simulink model "Model_14Bus_Microgrid_paper_Latam"  (R2022b)
settings: Solver=VariableStepAuto  StartTime=0.0  StopTime=0.5  MaxStep=1e-2  RelTol=1e-3
InitFcn:
  | Set_parameters_R2018
StopFcn:
  | %Save_Data;
  | %Graphics_mod;
values from neighbouring files (symbols this model uses):
  Clink = Ceq*2    (= 0.217013888889)    [Set_parameters.m]
  dis1 = 0.15    [Set_parameters.m]
  dis10 = 6    [Set_parameters.m]
  dis11 = 3    [Set_parameters.m]
  dis12 = 6    [Set_parameters.m]
  dis13 = 3    [Set_parameters.m]
  dis14 = 2    [Set_parameters.m]
  dis2 = 0.2    [Set_parameters.m]
  dis3 = 0.15    [Set_parameters.m]
  dis4 = 0.4    [Set_parameters.m]
  dis5 = 0.4    [Set_parameters.m]
  dis6 = 0.4    [Set_parameters.m]
  dis7 = 0.1    [Set_parameters.m]
  dis8 = 2    [Set_parameters.m]
  dis9 = 6    [Set_parameters.m]
  Fc = 33 * Fnom    (= 1980)    [Set_parameters.m]
  Fnom = 60    [Set_parameters.m]
  Increment_MPPT = 0.01    [Set_parameters.m]
  Ki_Ireg = 20    [Set_parameters.m]
  Ki_VDCreg = 400    [Set_parameters.m]
  Kp_Ireg = 0.3    [Set_parameters.m]
  Kp_VDCreg = 2    [Set_parameters.m]
  LimitL_Ireg = -1.5    [Set_parameters.m]
  LimitL_VDCreg = -1.5    [Set_parameters.m]
  Limits_MPPT = [ 583 357 ]    [Set_parameters.m]
  LimitU_Ireg = 1.5    [Set_parameters.m]
  LimitU_VDCreg = 1.5    [Set_parameters.m]
  P_Load_2 = S_Load_2* PF_Load_2    (= 36000)    [Set_parameters.m]
  P_Load_3 = S_Load_3* PF_Load_3    (= 25500)    [Set_parameters.m]
  Pnom = 1e6    (= 1000000)    [Set_parameters.m]
  Pnom_T1 = 1.5e6    (= 1500000)    [Set_parameters.m]
  Pnom_T2 = 1.5e6    (= 1500000)    [Set_parameters.m]
  Pnom_T3 = 4e6    (= 4000000)    [Set_parameters.m]
  Pnom_xfo = Pnom    (= 1000000)    [Set_parameters.m]
  Ql_Load_2 = S_Load_2 * sin(acos(PF_Load_2))    [Set_parameters.m]
  Ql_Load_3 = S_Load_3 * sin(acos(PF_Load_3))    [Set_parameters.m]
  R_Load_9 = (Vnom_prim * 1.35)^2 / P_Load_9    (= 1084.6153125)    [Set_parameters.m]
  R_Load_DC = Vnom_DC^2/ P_Load_DC    (= 45)    [Set_parameters.m]
  Rl = 0.394    [Set_parameters.m]
  Rls = 0.198    [Set_parameters.m]
  Ts = Ts_Power    (= 5.05050505051e-06)    [Set_parameters.m]
  Ts_Control = 10*Ts_Power    (= 5.05050505051e-05)    [Set_parameters.m]
  Ts_Power = 1/(33*Fnom)/100    (= 5.05050505051e-06)    [Set_parameters.m]
  V1_LL_T3 = 69e3    (= 69000)    [Set_parameters.m]
  Vf = 0    [Set_parameters.m]
  Vfd = 0    [Set_parameters.m]
  Vnom_dc = 480    [Set_parameters.m]
  Vnom_Diesel = 2.4e3    (= 2400)    [Set_parameters.m]
  Vnom_prim = 13.8e3    (= 13800)    [Set_parameters.m]
  Vnom_sec = 220    [Set_parameters.m]
  Vnom_ter_AC_DC = 150    [Set_parameters.m]
  Xl = 0.1168    [Set_parameters.m]
  Xls = 0.1089    [Set_parameters.m]
undefined symbols (not defined in the file or in its folder): D1, Delta, DiscIntNeverNeededParam, Hydride, Ion, level, Lithium, max_min, Metal, Nickel, RL, RLff, sigbuilder_block
libraries: spsRMSLib x73, powerlib_extras x53, spsCurrentMeasurementLib x47, spsTHDLib x26, spsThreePhaseVIMeasurementLib x25, spsVoltageMeasurementLib x23, spsSeriesRLCBranchLib x21, spsThreePhaseSeriesRLCBranchLib x21, spsIGBTDiodeLib x15, spsThreePhaseBreakerLib x14, spsPowerLib x14, spsThreePhaseTransformerTwoWindingsLib x12
(part 8 of 10)

== system Model_14Bus_Microgrid_paper_Latam/Bus_9/PLL/Pll3 ==
  note: error
  note: d'
  note: Fundamental
  note: fase
      | total
  note: fase de la señal
  note: adelanta 90
  note: Este PLL calcula la fase respecto a una onda coseno
  señal : Inport
  w : Inport  Port=2
  Gain : Gain  Gain=-1  SaturateOnIntegerOverflow=on  OutDataTypeStr=Inherit: Same as input  ParamDataTypeStr=Inherit: Same as input
  Integrator : Integrator  InitialCondition=2*pi*60
  Integrator1 : Integrator  InitialCondition=2*pi*60
  Integrator2 : Integrator
  K : Gain  Gain=100  SaturateOnIntegerOverflow=on  OutDataTypeStr=Inherit: Same as input  ParamDataTypeStr=Inherit: Same as input
  Kp : Gain  Gain=10  SaturateOnIntegerOverflow=on  OutDataTypeStr=Inherit: Same as input  ParamDataTypeStr=Inherit: Same as input
  Kp1 : Gain  Gain=10  SaturateOnIntegerOverflow=on  OutDataTypeStr=Inherit: Same as input  ParamDataTypeStr=Inherit: Same as input
  Poduct : Product  SaturateOnIntegerOverflow=on  OutDataTypeStr=Inherit: Same as first input
  Poduct1 : Product  SaturateOnIntegerOverflow=on  OutDataTypeStr=Inherit: Same as first input
  Poduct2 : Product  SaturateOnIntegerOverflow=on  OutDataTypeStr=Inherit: Same as first input
  Sum : Sum  Inputs=|+-  SaturateOnIntegerOverflow=on
  Sum1 : Sum  SaturateOnIntegerOverflow=on
  Sum2 : Sum  Inputs=|-+  SaturateOnIntegerOverflow=on
  Trigonometric Function : Trigonometry
  Trigonometric Function1 : Trigonometry  Operator=cos
  f cos (rad) : Outport  VectorParamsAs1DForOutWhenUnconnected=off
  wires:
  Sum/1 -> Poduct/1, Poduct1/1
  Poduct/1 -> Kp/1
  Kp/1 -> Kp1/1
  Poduct2/1 -> Sum/2
  Trigonometric Function1/1 -> Poduct1/2, Poduct2/1
  Poduct1/1 -> K/1
  K/1 -> Integrator2/1
  Integrator2/1 -> Poduct2/2
  Integrator/1 -> Trigonometric Function/1, Sum2/2, Trigonometric Function1/1
  Integrator1/1 -> Sum2/1
  Sum2/1 -> f cos (rad)/1
  w/1 -> Sum1/1, Integrator1/1
  Kp1/1 -> Sum1/2
  Sum1/1 -> Integrator/1
  Trigonometric Function/1 -> Gain/1
  Gain/1 -> Poduct/2
  señal/1 -> Sum/1

== system Model_14Bus_Microgrid_paper_Latam/Bus_slack /PLL/Pll1 ==
  note: error
  note: d'
  note: Fundamental
  note: fase
      | total
  note: fase de la señal
  note: adelanta 90
  note: Este PLL calcula la fase respecto a una onda coseno
  señal : Inport
  w : Inport  Port=2
  Gain : Gain  Gain=-1  SaturateOnIntegerOverflow=on  OutDataTypeStr=Inherit: Same as input  ParamDataTypeStr=Inherit: Same as input
  Integrator : Integrator  InitialCondition=2*pi*60
  Integrator1 : Integrator  InitialCondition=2*pi*60
  Integrator2 : Integrator
  K : Gain  Gain=100  SaturateOnIntegerOverflow=on  OutDataTypeStr=Inherit: Same as input  ParamDataTypeStr=Inherit: Same as input
  Kp : Gain  Gain=10  SaturateOnIntegerOverflow=on  OutDataTypeStr=Inherit: Same as input  ParamDataTypeStr=Inherit: Same as input
  Kp1 : Gain  Gain=10  SaturateOnIntegerOverflow=on  OutDataTypeStr=Inherit: Same as input  ParamDataTypeStr=Inherit: Same as input
  Poduct : Product  SaturateOnIntegerOverflow=on  OutDataTypeStr=Inherit: Same as first input
  Poduct1 : Product  SaturateOnIntegerOverflow=on  OutDataTypeStr=Inherit: Same as first input
  Poduct2 : Product  SaturateOnIntegerOverflow=on  OutDataTypeStr=Inherit: Same as first input
  Sum : Sum  Inputs=|+-  SaturateOnIntegerOverflow=on
  Sum1 : Sum  SaturateOnIntegerOverflow=on
  Sum2 : Sum  Inputs=|-+  SaturateOnIntegerOverflow=on
  Trigonometric Function : Trigonometry
  Trigonometric Function1 : Trigonometry  Operator=cos
  f cos (rad) : Outport  VectorParamsAs1DForOutWhenUnconnected=off
  wires:
  Sum/1 -> Poduct/1, Poduct1/1
  Poduct/1 -> Kp/1
  Kp/1 -> Kp1/1
  Poduct2/1 -> Sum/2
  Trigonometric Function1/1 -> Poduct1/2, Poduct2/1
  Poduct1/1 -> K/1
  K/1 -> Integrator2/1
  Integrator2/1 -> Poduct2/2
  Integrator/1 -> Trigonometric Function/1, Sum2/2, Trigonometric Function1/1
  Integrator1/1 -> Sum2/1
  Sum2/1 -> f cos (rad)/1
  w/1 -> Sum1/1, Integrator1/1
  Kp1/1 -> Sum1/2
  Sum1/1 -> Integrator/1
  Trigonometric Function/1 -> Gain/1
  Gain/1 -> Poduct/2
  señal/1 -> Sum/1

== system Model_14Bus_Microgrid_paper_Latam/Bus_slack /PLL/Pll2 ==
  note: error
  note: d'
  note: Fundamental
  note: fase
      | total
  note: fase de la señal
  note: adelanta 90
  note: Este PLL calcula la fase respecto a una onda coseno
  señal : Inport
  w : Inport  Port=2
  Gain : Gain  Gain=-1  SaturateOnIntegerOverflow=on  OutDataTypeStr=Inherit: Same as input  ParamDataTypeStr=Inherit: Same as input
  Integrator : Integrator  InitialCondition=2*pi*60
  Integrator1 : Integrator  InitialCondition=2*pi*60
  Integrator2 : Integrator
  K : Gain  Gain=100  SaturateOnIntegerOverflow=on  OutDataTypeStr=Inherit: Same as input  ParamDataTypeStr=Inherit: Same as input
  Kp : Gain  Gain=10  SaturateOnIntegerOverflow=on  OutDataTypeStr=Inherit: Same as input  ParamDataTypeStr=Inherit: Same as input
  Kp1 : Gain  Gain=10  SaturateOnIntegerOverflow=on  OutDataTypeStr=Inherit: Same as input  ParamDataTypeStr=Inherit: Same as input
  Poduct : Product  SaturateOnIntegerOverflow=on  OutDataTypeStr=Inherit: Same as first input
  Poduct1 : Product  SaturateOnIntegerOverflow=on  OutDataTypeStr=Inherit: Same as first input
  Poduct2 : Product  SaturateOnIntegerOverflow=on  OutDataTypeStr=Inherit: Same as first input
  Sum : Sum  Inputs=|+-  SaturateOnIntegerOverflow=on
  Sum1 : Sum  SaturateOnIntegerOverflow=on
  Sum2 : Sum  Inputs=|-+  SaturateOnIntegerOverflow=on
  Trigonometric Function : Trigonometry
  Trigonometric Function1 : Trigonometry  Operator=cos
  f cos (rad) : Outport  VectorParamsAs1DForOutWhenUnconnected=off
  wires:
  Sum/1 -> Poduct/1, Poduct1/1
  Poduct/1 -> Kp/1
  Kp/1 -> Kp1/1
  Poduct2/1 -> Sum/2
  Trigonometric Function1/1 -> Poduct1/2, Poduct2/1
  Poduct1/1 -> K/1
  K/1 -> Integrator2/1
  Integrator2/1 -> Poduct2/2
  Integrator/1 -> Trigonometric Function/1, Sum2/2, Trigonometric Function1/1
  Integrator1/1 -> Sum2/1
  Sum2/1 -> f cos (rad)/1
  w/1 -> Sum1/1, Integrator1/1
  Kp1/1 -> Sum1/2
  Sum1/1 -> Integrator/1
  Trigonometric Function/1 -> Gain/1
  Gain/1 -> Poduct/2
  señal/1 -> Sum/1

== system Model_14Bus_Microgrid_paper_Latam/Bus_slack /PLL/Pll3 ==
  note: error
  note: d'
  note: Fundamental
  note: fase
      | total
  note: fase de la señal
  note: adelanta 90
  note: Este PLL calcula la fase respecto a una onda coseno
  señal : Inport
  w : Inport  Port=2
  Gain : Gain  Gain=-1  SaturateOnIntegerOverflow=on  OutDataTypeStr=Inherit: Same as input  ParamDataTypeStr=Inherit: Same as input
  Integrator : Integrator  InitialCondition=2*pi*60
  Integrator1 : Integrator  InitialCondition=2*pi*60
  Integrator2 : Integrator
  K : Gain  Gain=100  SaturateOnIntegerOverflow=on  OutDataTypeStr=Inherit: Same as input  ParamDataTypeStr=Inherit: Same as input
  Kp : Gain  Gain=10  SaturateOnIntegerOverflow=on  OutDataTypeStr=Inherit: Same as input  ParamDataTypeStr=Inherit: Same as input
  Kp1 : Gain  Gain=10  SaturateOnIntegerOverflow=on  OutDataTypeStr=Inherit: Same as input  ParamDataTypeStr=Inherit: Same as input
  Poduct : Product  SaturateOnIntegerOverflow=on  OutDataTypeStr=Inherit: Same as first input
  Poduct1 : Product  SaturateOnIntegerOverflow=on  OutDataTypeStr=Inherit: Same as first input
  Poduct2 : Product  SaturateOnIntegerOverflow=on  OutDataTypeStr=Inherit: Same as first input
  Sum : Sum  Inputs=|+-  SaturateOnIntegerOverflow=on
  Sum1 : Sum  SaturateOnIntegerOverflow=on
  Sum2 : Sum  Inputs=|-+  SaturateOnIntegerOverflow=on
  Trigonometric Function : Trigonometry
  Trigonometric Function1 : Trigonometry  Operator=cos
  f cos (rad) : Outport  VectorParamsAs1DForOutWhenUnconnected=off
  wires:
  Sum/1 -> Poduct/1, Poduct1/1
  Poduct/1 -> Kp/1
  Kp/1 -> Kp1/1
  Poduct2/1 -> Sum/2
  Trigonometric Function1/1 -> Poduct1/2, Poduct2/1
  Poduct1/1 -> K/1
  K/1 -> Integrator2/1
  Integrator2/1 -> Poduct2/2
  Integrator/1 -> Trigonometric Function/1, Sum2/2, Trigonometric Function1/1
  Integrator1/1 -> Sum2/1
  Sum2/1 -> f cos (rad)/1
  w/1 -> Sum1/1, Integrator1/1
  Kp1/1 -> Sum1/2
  Sum1/1 -> Integrator/1
  Trigonometric Function/1 -> Gain/1
  Gain/1 -> Poduct/2
  señal/1 -> Sum/1

== system Model_14Bus_Microgrid_paper_Latam/Line 13 (3km)/Load_4/Power Factor Block1 ==
  Vabc : Inport
  Iabc : Inport  Port=2
  Complex to Magnitude-Angle : ComplexToMagnitudeAngle
  Mux : Mux  Inputs=2
  Mux1 : Mux  Inputs=2
  Power : spsPowerLib/Power  Freq=Freq  Vinit=Vinit  Iinit=Iinit  Ts=Ts
  RMS3 : spsRMSLib/RMS  TrueRMS=on  Freq=60  RMSInit=0  Ts=0
  RMS4 : spsRMSLib/RMS  TrueRMS=on  Freq=60  RMSInit=0  Ts=0
  Real-Imag to Complex : RealImagToComplex
  Terminator : Terminator
  compara : Gain  SaturateOnIntegerOverflow=on  OutDataTypeStr=Inherit: Same as input  ParamDataTypeStr=Inherit: Same as input
  cos(theta) : Trigonometry  Operator=cos
  Pabc : Outport  VectorParamsAs1DForOutWhenUnconnected=off
  Qabc : Outport  Port=2  VectorParamsAs1DForOutWhenUnconnected=off
  Vabc y Vabc (rms) : Outport  Port=3  VectorParamsAs1DForOutWhenUnconnected=off
  Iabc y Iabc (rms) : Outport  Port=4  VectorParamsAs1DForOutWhenUnconnected=off
  "PFabc " : Outport  Port=5  VectorParamsAs1DForOutWhenUnconnected=off
  wires:
  Power/1 -> Pabc/1, Real-Imag to Complex/1
  Power/2 -> Qabc/1, Real-Imag to Complex/2
  Complex to Magnitude-Angle/2 -> cos(theta)/1
  Real-Imag to Complex/1 -> Complex to Magnitude-Angle/1
  cos(theta)/1 -> "PFabc "/1
  Complex to Magnitude-Angle/1 -> Terminator/1
  Iabc/1 -> RMS4/1, compara/1, Power/2
  RMS4/1 -> Mux1/2
  Mux1/1 -> Iabc y Iabc (rms)/1
  Mux/1 -> Vabc y Vabc (rms)/1
  Vabc/1 -> Power/1, Mux/2, RMS3/1
  compara/1 -> Mux1/1
  RMS3/1 -> Mux/1

== system Model_14Bus_Microgrid_paper_Latam/Solar PV /Inversor PV 480 // 250 DC // AC /Control de inversor ==
  On : Inport  PortDimensions=1
  Vabc_prim : Inport  Port=2  PortDimensions=3
  Iabc_prim : Inport  Port=3  PortDimensions=3
  Vdc_meas : Inport  Port=4  PortDimensions=1
  V_PV : Inport  Port=5  PortDimensions=1
  I_PV : Inport  Port=6  PortDimensions=1
  Current Regulator : Subsystem
  Iq_ref : Constant  Value=0
  MPPT Parameters : Subsystem
  "MPPT Controller using Perturbe & Observe technique " : MATLAB Function  TreatAsAtomicUnit=on
  Mux : Mux  Inputs=2
  Overmodulation : spsOvermodulationLib/Overmodulation  OverModType=Flat top
      settings: LibrarySourceBlock=sps_lib/Power Electronics/Power Electronics Control/Overmodulation
  PLL & Measurements : Subsystem
  PWM Generator (3-Level) : spsPWMGenerator3LevelLib/PWM Generator (3-Level)  ModulatorType=Three-phase bridge (12 pulses)  ModulatorMode=Unsynchronized  nF=27  Fc=Fc  ModulatingSignals=off  m=0.8  Freq=60  Phase=0  Ts=Ts_PWMgenerator
      settings: LibrarySourceBlock=|
      | sps_lib/Power Electronics/Power Electronics Control/PWM Generator
      | (3-Level)
  Switch : Switch  Criteria=u2 ~= 0  SaturateOnIntegerOverflow=off  InputSameDT=off
  Uabc_ref Generation max (m) = 1 : Subsystem
  Unit Delay : UnitDelay  SampleTime=Ts_Control  HasFrameUpgradeWarning=on
  VDC Regulator : Subsystem
  Vnom_dc1 : Constant  Value=Vdc_ref_Init
  g : Outport  VectorParamsAs1DForOutWhenUnconnected=off
  tag scope: Id_ref=global, Uref1=global, Uref2=global, Vdc_ref=global
  wires:
  PLL & Measurements/1(wt) -> Uabc_ref Generation max (m) = 1/1(wt)
  Current Regulator/1(VdVq_conv) -> Uabc_ref Generation max (m) = 1/2(VdVq_conv)
  Iq_ref/1 -> Mux/2
  Mux/1 -> Current Regulator/3(IdIq_ref)
  PLL & Measurements/3(IdIq_prim) -> Current Regulator/2(IdIq_meas)
  PLL & Measurements/2(VdVq_prim) -> Current Regulator/1(VdVq_meas)
  Vabc_prim/1 -> PLL & Measurements/1(Vabc_prim)
  Iabc_prim/1 -> PLL & Measurements/2(Iabc_prim)
  PWM Generator (3-Level)/1 -> g/1
  Vdc_meas/1 -> VDC Regulator/1(Vdc_meas)
  VDC Regulator/1(Id_ref) -> [Id_ref], Mux/1
  V_PV/1 -> "MPPT Controller using Perturbe & Observe technique "/3(V)
  I_PV/1 -> "MPPT Controller using Perturbe & Observe technique "/4(I)
  MPPT Parameters/1(Param) -> "MPPT Controller using Perturbe & Observe technique "/1(Param)
  On/1 -> "MPPT Controller using Perturbe & Observe technique "/2(Enabled), Switch/2
  Overmodulation/1 -> [Uref2], PWM Generator (3-Level)/1
  Unit Delay/1 -> [Uref1], Overmodulation/1
  "MPPT Controller using Perturbe & Observe technique "/1(D) -> Switch/1
  Switch/1 -> [Vdc_ref], VDC Regulator/2(Vdc_ref)
  Vnom_dc1/1 -> Switch/3
  Uabc_ref Generation max (m) = 1/1(Uabc_ref) -> Unit Delay/1

== system Model_14Bus_Microgrid_paper_Latam/Solar PV /Recurso solar/Irradiancia Temp Demand Max ==
  Demux : Demux  Tag=STV Demux  Outputs=2
      settings: DisplayOption=none
  FromWs : FromWorkspace  Tag=STV FromWs  VariableName=tuvar
      SigBuilderData=|
      | common.afterFinalStr = 'Extrapolate'
      | common.sampleTime = '0'
      | dataSet(1).timeRange = [0 2]
      | dataSet(1).name = 'Constant Irradiance'
      | dataSet(2).timeRange = [0 2]
      | dataSet(2).name = 'Step Irradiance'
      | dataSet(3).timeRange = [0 3]
      | dataSet(3).name = 'Ramp-up/down Irradiance'
      | sbobj.Groups(1).Name = 'Constant Irradiance'
      | sbobj.Groups(1).Signals(1).Name = 'Ir'
      | sbobj.Groups(1).Signals(1).XData = [0 2]
      | sbobj.Groups(1).Signals(1).YData = [1000 1000]
      | sbobj.Groups(1).Signals(2).Name = 'Temp'
      | sbobj.Groups(1).Signals(2).XData = [0 1 1 2]
      | sbobj.Groups(1).Signals(2).YData = [0 0 1 1]
      | sbobj.Groups(1).TimeRange = [0 2]
      | sbobj.Groups(2).Name = 'Step Irradiance'
      | sbobj.Groups(2).Signals(1).Name = 'Ir'
      | sbobj.Groups(2).Signals(1).XData = [0 0.252 0.252 2]
      | sbobj.Groups(2).Signals(1).YData = [600 600 1000 1000]
      | sbobj.Groups(2).Signals(2).Name = 'Temp'
      | sbobj.Groups(2).Signals(2).XData = [0 1 1 2]
      | sbobj.Groups(2).Signals(2).YData = [0 0 1 1]
      | sbobj.Groups(2).TimeRange = [0 2]
      | sbobj.Groups(3).Name = 'Ramp-up/down Irradiance'
      | sbobj.Groups(3).Signals(1).Name = 'Ir'
      | sbobj.Groups(3).Signals(1).XData = [0 0.785 1.7 2.28 3]
      | sbobj.Groups(3).Signals(1).YData = [1000 999.538235294 999 999.446153846 1000]
      | sbobj.Groups(3).Signals(2).Name = 'Temp'
      | sbobj.Groups(3).Signals(2).XData = [0 2 2.1 3]
      | sbobj.Groups(3).Signals(2).YData = [25 25 25 25]
      | sbobj.Groups(3).TimeRange = [0 3]
  Ir : Outport  Tag=STV Outport  VectorParamsAs1DForOutWhenUnconnected=off
  Temp : Outport  Tag=STV Outport  Port=2  VectorParamsAs1DForOutWhenUnconnected=off
  wires:
  Demux/1 -> Ir/1
  FromWs/1 -> Demux/1
  Demux/2 -> Temp/1

== system Model_14Bus_Microgrid_paper_Latam/Subsystem1/Bus_AC//DC4/PLL ==
  Vabc_LN_pu : Inport
  2pi60'1 : Constant  Value=2*pi*60
  2pi60'2 : Constant  Value=2*pi*60
  2pi60'3 : Constant  Value=2*pi*60
  Constant : Constant  Value=90
  Demux : Demux  Outputs=3
  Gain1 : Gain  Gain=180/pi  SaturateOnIntegerOverflow=on  OutDataTypeStr=Inherit: Same as input  ParamDataTypeStr=Inherit: Same as input
  Gain2 : Gain  Gain=180/pi  SaturateOnIntegerOverflow=on  OutDataTypeStr=Inherit: Same as input  ParamDataTypeStr=Inherit: Same as input
  Gain3 : Gain  Gain=180/pi  SaturateOnIntegerOverflow=on  OutDataTypeStr=Inherit: Same as input  ParamDataTypeStr=Inherit: Same as input
  Mux : Mux  Inputs=3
  Pll1 : Subsystem
  Pll2 : Subsystem
  Pll3 : Subsystem
  Sum : Sum  Inputs=|++
  delta_abc : Outport  VectorParamsAs1DForOutWhenUnconnected=off
  wires:
  Vabc_LN_pu/1 -> Demux/1
  Demux/1 -> Pll3/1(señal)
  2pi60'3/1 -> Pll3/2(w)
  Pll3/1(f cos (rad)) -> Gain1/1
  Demux/2 -> Pll1/1(señal)
  2pi60'1/1 -> Pll1/2(w)
  Gain2/1 -> Mux/2
  Demux/3 -> Pll2/1(señal)
  2pi60'2/1 -> Pll2/2(w)
  Pll2/1(f cos (rad)) -> Gain3/1
  Gain3/1 -> Mux/3
  Pll1/1(f cos (rad)) -> Gain2/1
  Mux/1 -> Sum/1
  Gain1/1 -> Mux/1
  Constant/1 -> Sum/2
  Sum/1 -> delta_abc/1

== system Model_14Bus_Microgrid_paper_Latam/Subsystem1/Bus_AC//DC4/Power Factor Block1 ==
  Vabc : Inport
  Iabc : Inport  Port=2
  Complex to Magnitude-Angle : ComplexToMagnitudeAngle
  Mux : Mux  Inputs=2
  Mux1 : Mux  Inputs=2
  Power : spsPowerLib/Power  Freq=Freq  Vinit=Vinit  Iinit=Iinit  Ts=Ts
  RMS3 : spsRMSLib/RMS  TrueRMS=on  Freq=60  RMSInit=0  Ts=0
  RMS4 : spsRMSLib/RMS  TrueRMS=on  Freq=60  RMSInit=0  Ts=0
  Real-Imag to Complex : RealImagToComplex
  Terminator : Terminator
  compara : Gain  SaturateOnIntegerOverflow=on  OutDataTypeStr=Inherit: Same as input  ParamDataTypeStr=Inherit: Same as input
  cos(theta) : Trigonometry  Operator=cos
  Pabc : Outport  VectorParamsAs1DForOutWhenUnconnected=off
  Qabc : Outport  Port=2  VectorParamsAs1DForOutWhenUnconnected=off
  Vabc y Vabc (rms) : Outport  Port=3  VectorParamsAs1DForOutWhenUnconnected=off
  Iabc y Iabc (rms) : Outport  Port=4  VectorParamsAs1DForOutWhenUnconnected=off
  "PFabc " : Outport  Port=5  VectorParamsAs1DForOutWhenUnconnected=off
  wires:
  Power/1 -> Pabc/1, Real-Imag to Complex/1
  Power/2 -> Qabc/1, Real-Imag to Complex/2
  Complex to Magnitude-Angle/2 -> cos(theta)/1
  Real-Imag to Complex/1 -> Complex to Magnitude-Angle/1
  cos(theta)/1 -> "PFabc "/1
  Complex to Magnitude-Angle/1 -> Terminator/1
  Iabc/1 -> RMS4/1, compara/1, Power/2
  RMS4/1 -> Mux1/2
  Mux1/1 -> Iabc y Iabc (rms)/1
  Mux/1 -> Vabc y Vabc (rms)/1
  Vabc/1 -> Power/1, Mux/2, RMS3/1
  compara/1 -> Mux1/1
  RMS3/1 -> Mux/1

== system Model_14Bus_Microgrid_paper_Latam/Subsystem1/Control measurement/measurement ==
  Ground4 : spsGroundLib/Ground  LConnTagsString=a
  Mux1 : Mux  Inputs=3
  Mux2 : Mux  Inputs=3
  Mux7 : Mux  Inputs=3
  Vab : spsVoltageMeasurementLib/Voltage Measurement  Tag=PoWeRsYsTeMmEaSuReMeNt  PhasorSimulation=off  OutputType=Magnitude  PSBequivalent=0
  Vab{1..3,5} (4 alike) : powerlib_extras/Discrete Measurements/Discrete  RMS value  Freq=60  Mag_Init=0  Ts=Ts_Power
  Vbc : spsVoltageMeasurementLib/Voltage Measurement  Tag=PoWeRsYsTeMmEaSuReMeNt  PhasorSimulation=off  OutputType=Magnitude  PSBequivalent=0
  Vca : spsVoltageMeasurementLib/Voltage Measurement  Tag=PoWeRsYsTeMmEaSuReMeNt  PhasorSimulation=off  OutputType=Magnitude  PSBequivalent=0
  a : spsVoltageMeasurementLib/Voltage Measurement  Tag=PoWeRsYsTeMmEaSuReMeNt  PhasorSimulation=off  OutputType=Magnitude  PSBequivalent=0
  b : spsVoltageMeasurementLib/Voltage Measurement  Tag=PoWeRsYsTeMmEaSuReMeNt  PhasorSimulation=off  OutputType=Magnitude  PSBequivalent=0
  c : spsVoltageMeasurementLib/Voltage Measurement  Tag=PoWeRsYsTeMmEaSuReMeNt  PhasorSimulation=off  OutputType=Magnitude  PSBequivalent=0
  A : PMIOPort  Side=Left
  B : PMIOPort  Port=2  Side=Left
  C : PMIOPort  Port=3  Side=Left
  Vph : Outport  VectorParamsAs1DForOutWhenUnconnected=off
  VL-L : Outport  Port=2  VectorParamsAs1DForOutWhenUnconnected=off
  VL-L_rms : Outport  Port=3  VectorParamsAs1DForOutWhenUnconnected=off
  Vph_rms : Outport  Port=4  VectorParamsAs1DForOutWhenUnconnected=off
  wires:
  a/1 -> Mux7/1, Vab5/1
  b/1 -> Mux7/2, Vab1/1
  c/1 -> Mux7/3, Vab2/1
  Mux7/1 -> Vph/1
  Vab/1 -> Mux1/1
  Vbc/1 -> Mux1/2
  Vca/1 -> Mux1/3
  Mux1/1 -> Vab3/1, VL-L/1
  Vab5/1 -> Mux2/1
  Vab1/1 -> Mux2/2
  Vab2/1 -> Mux2/3
  Mux2/1 -> Vph_rms/1
  Vab3/1 -> VL-L_rms/1
  connections:
  Ground4/LConn1 -- c/LConn2 -- b/LConn2 -- a/LConn2
  A/RConn1 -- a/LConn1 -- Vab/LConn1 -- Vca/LConn2
  B/RConn1 -- b/LConn1 -- Vab/LConn2 -- Vbc/LConn1
  C/RConn1 -- c/LConn1 -- Vbc/LConn2 -- Vca/LConn1

== system Model_14Bus_Microgrid_paper_Latam/Subsystem1/Convertidor bidireccional 1.1 300 (DC) // 150 V (AC) P_nom 3kW/Control of Inverter ==
  note: VL-L rms_1
  note: Primary control
  note: Control of Inverter
  Means : Inport
  Bus Selector : BusSelector  OutputSignals=signal1,signal2,signal3,signal4
  Discrete PWM Generator1 : Subsystem  AncestorBlock=|  DialogController=POWERSYS.PowerSysDialog  mask(Discrete PWM Generator){GeneratorMode=3-arm  bridge (6 pulses), Fc=4000, Ts=Ts_Power, Internal=off, mIndex=0.99, Freq=60, Phase=0}
      | powerlib_extras/Discrete 
      | Control Blocks/Discrete
      | PWM Generator
      mask prompts: GeneratorMode "Generator Mode"; Fc "Carrier frequency (Hz):"; Ts "Sample time:"; Internal "Internal generation of modulating signal(s)"; mIndex "Modulation index  (0<m<1) :"; Freq "Frequency of output voltage (Hz)"; Phase "Phase of output voltage (degrees)"
      mask help:
      | This discrete block generates pulses for carrier-based PWM (Pulse Width Modulation), self-commutated IGBTs,GTOs or FETs bridges.
      |
      | Depending on the number of bridge arms selected in the "Generator Mode" parameter, the block can be used either for single-phase or three-phase PWM control.
      mask init:
      | powericon('psbcallbacks',gcb,'Discrete PWM Generator');
      | if Freq==0
      |     Phase=90;
      | end
      | switch GeneratorMode
      | case 1,
      |     Internal_Phase=0;
      |    Signal_PortWidth=1;
      |    Select1_Elements=[1 2];
      |    Select1_PortWidth=2;
      |    Select3_Elements=[1 2];
      |    Select3_PortWidth=4;
      | case 2,
      |     Internal_Phase=0;
      |     Signal_PortWidth=1;
      |     Select1_Elements=[1 2];
      |     Select1_PortWidth=2;
      |     Select3_Elements=[1 2 3 4];
      |     Select3_PortWidth=4;
      | case 3,
      |     Internal_Phase=[0 -2*pi/3 2*pi/3];
      |     Signal_PortWidth=3;
      |     Select1_Elements=[1 4 2 5 3 6];
      |     Select1_PortWidth=6;
      |    Select3_Elements=[1 2 3 4 5 6];
      |    Select3_PortWidth=12;
      | case 4,
      |     Internal_Phase=[0 -2*pi/3 2*pi/3];
      |     Signal_PortWidth=3;
      |     Select1_Elements=[1 4 2 5 3 6];
      |     Select1_PortWidth=6;
      |    Select3_Elements=[1 2 3 4 5 6 7 8 9 10 11 12];
      |    Select3_PortWidth=12;
      | end
      | power_initmask();
      settings: LibrarySourceBlock=|
      | powerlib_extras/Discrete
      | Control Blocks/Discrete
      | PWM Generator
      mask Help:
      | The output pulses are a vector (with values=0 or 1). Depending on the selected "Generator Mode", the output vector contains:
      | For a 1-arm  bridge: Two pulses. Pulse 1 is for the upper switch and pulse 2 is for the lower switch.
      | For a 2-arm  bridge: Four pulses. Pulses 1 and 3 are respectively for the upper switches of the first and second arm. Pulses 2 and 4 are for the lower switches.
      | For a 3-arm  bridge: Six pulses. Pulses 1,3 and 5 are respectively for the upper switches of the first,second and third arm. Pulses 2,4 and 6 are for the lower switches.
      | For double 3-arm bridges: Twelve pulses.The first six pulses (pulses 1 to 6) must be sent to the first 3-arm bridge and the last six (pulses 7 to 12) to the second 3-arm bridge.
      | 
      | By selecting "Internal generation" you can can control the modulation index m, frequency and phase of the output voltage  from the internal parameters (m, Freq and Phase). Otherwise, external signals are used for pulse generation. The width of the input vector must be 1 for single phase bridges ( 1-arm or 2-arm)  and 3 for 3-phase bridges  (single or double bridge).
      mask TypeOptions GeneratorMode: 1-arm  bridge (2 pulses) | 2-arm  bridge (4 pulses) | 3-arm  bridge (6 pulses) | Double 3-arm  bridges (12 pulses)
      mask Callback Internal: powericon('psbcallbacks',gcb,'Discrete PWM Generator',[]);
  MI Controller : Subsystem
  Unit Delay4 : UnitDelay  SampleTime=Ts_Power  HasFrameUpgradeWarning=on
  VL-L_1 : Scope  NumInputPorts=2
  Vph_abc : Scope
  Vph_rms_1 : Scope
  u / m : Scope
  Pulses : Outport  VectorParamsAs1DForOutWhenUnconnected=off
  wires:
  MI Controller/2(u / m) -> u / m/1
  Unit Delay4/1 -> Pulses/1
  Discrete PWM Generator1/1(Pulses) -> Unit Delay4/1
  Bus Selector/1 -> Vph_abc/1, MI Controller/1(Vabc)  "<signal1>"
  Bus Selector/2 -> VL-L_1/1  "<signal2>"
  Bus Selector/3 -> VL-L_1/2  "<signal3>"
  Bus Selector/4 -> Vph_rms_1/1  "<signal4>"
  Means/1 -> Bus Selector/1
  MI Controller/1(Vabc_inv) -> Discrete PWM Generator1/1(Uref)

== system Model_14Bus_Microgrid_paper_Latam/Subsystem3/Bus_AC//DC5/PLL ==
  Vabc_LN_pu : Inport
  2pi60'1 : Constant  Value=2*pi*60
  2pi60'2 : Constant  Value=2*pi*60
  2pi60'3 : Constant  Value=2*pi*60
  Constant : Constant  Value=90
  Demux : Demux  Outputs=3
  Gain1 : Gain  Gain=180/pi  SaturateOnIntegerOverflow=on  OutDataTypeStr=Inherit: Same as input  ParamDataTypeStr=Inherit: Same as input
  Gain2 : Gain  Gain=180/pi  SaturateOnIntegerOverflow=on  OutDataTypeStr=Inherit: Same as input  ParamDataTypeStr=Inherit: Same as input
  Gain3 : Gain  Gain=180/pi  SaturateOnIntegerOverflow=on  OutDataTypeStr=Inherit: Same as input  ParamDataTypeStr=Inherit: Same as input
  Mux : Mux  Inputs=3
  Pll1 : Subsystem
  Pll2 : Subsystem
  Pll3 : Subsystem
  Sum : Sum  Inputs=|++
  delta_abc : Outport  VectorParamsAs1DForOutWhenUnconnected=off
  wires:
  Vabc_LN_pu/1 -> Demux/1
  Demux/1 -> Pll3/1(señal)
  2pi60'3/1 -> Pll3/2(w)
  Pll3/1(f cos (rad)) -> Gain1/1
  Demux/2 -> Pll1/1(señal)
  2pi60'1/1 -> Pll1/2(w)
  Gain2/1 -> Mux/2
  Demux/3 -> Pll2/1(señal)
  2pi60'2/1 -> Pll2/2(w)
  Pll2/1(f cos (rad)) -> Gain3/1
  Gain3/1 -> Mux/3
  Pll1/1(f cos (rad)) -> Gain2/1
  Mux/1 -> Sum/1
  Gain1/1 -> Mux/1
  Constant/1 -> Sum/2
  Sum/1 -> delta_abc/1

== system Model_14Bus_Microgrid_paper_Latam/Subsystem3/Bus_AC//DC5/Power Factor Block1 ==
  Vabc : Inport
  Iabc : Inport  Port=2
  Complex to Magnitude-Angle : ComplexToMagnitudeAngle
  Mux : Mux  Inputs=2
  Mux1 : Mux  Inputs=2
  Power : spsPowerLib/Power  Freq=Freq  Vinit=Vinit  Iinit=Iinit  Ts=Ts
  RMS3 : spsRMSLib/RMS  TrueRMS=on  Freq=60  RMSInit=0  Ts=0
  RMS4 : spsRMSLib/RMS  TrueRMS=on  Freq=60  RMSInit=0  Ts=0
  Real-Imag to Complex : RealImagToComplex
  Terminator : Terminator
  compara : Gain  SaturateOnIntegerOverflow=on  OutDataTypeStr=Inherit: Same as input  ParamDataTypeStr=Inherit: Same as input
  cos(theta) : Trigonometry  Operator=cos
  Pabc : Outport  VectorParamsAs1DForOutWhenUnconnected=off
  Qabc : Outport  Port=2  VectorParamsAs1DForOutWhenUnconnected=off
  Vabc y Vabc (rms) : Outport  Port=3  VectorParamsAs1DForOutWhenUnconnected=off
  Iabc y Iabc (rms) : Outport  Port=4  VectorParamsAs1DForOutWhenUnconnected=off
  "PFabc " : Outport  Port=5  VectorParamsAs1DForOutWhenUnconnected=off
  wires:
  Power/1 -> Pabc/1, Real-Imag to Complex/1
  Power/2 -> Qabc/1, Real-Imag to Complex/2
  Complex to Magnitude-Angle/2 -> cos(theta)/1
  Real-Imag to Complex/1 -> Complex to Magnitude-Angle/1
  cos(theta)/1 -> "PFabc "/1
  Complex to Magnitude-Angle/1 -> Terminator/1
  Iabc/1 -> RMS4/1, compara/1, Power/2
  RMS4/1 -> Mux1/2
  Mux1/1 -> Iabc y Iabc (rms)/1
  Mux/1 -> Vabc y Vabc (rms)/1
  Vabc/1 -> Power/1, Mux/2, RMS3/1
  compara/1 -> Mux1/1
  RMS3/1 -> Mux/1

== system Model_14Bus_Microgrid_paper_Latam/Subsystem3/Control measurement2/measurement2 ==
  Ground4 : spsGroundLib/Ground  LConnTagsString=a
  Mux1 : Mux  Inputs=3
  Mux2 : Mux  Inputs=3
  Mux7 : Mux  Inputs=3
  Vab : spsVoltageMeasurementLib/Voltage Measurement  Tag=PoWeRsYsTeMmEaSuReMeNt  PhasorSimulation=off  OutputType=Magnitude  PSBequivalent=0
  Vab{1..3,5} (4 alike) : powerlib_extras/Discrete Measurements/Discrete  RMS value  Freq=60  Mag_Init=0  Ts=Ts_Power
  Vbc : spsVoltageMeasurementLib/Voltage Measurement  Tag=PoWeRsYsTeMmEaSuReMeNt  PhasorSimulation=off  OutputType=Magnitude  PSBequivalent=0
  Vca : spsVoltageMeasurementLib/Voltage Measurement  Tag=PoWeRsYsTeMmEaSuReMeNt  PhasorSimulation=off  OutputType=Magnitude  PSBequivalent=0
  a : spsVoltageMeasurementLib/Voltage Measurement  Tag=PoWeRsYsTeMmEaSuReMeNt  PhasorSimulation=off  OutputType=Magnitude  PSBequivalent=0
  b : spsVoltageMeasurementLib/Voltage Measurement  Tag=PoWeRsYsTeMmEaSuReMeNt  PhasorSimulation=off  OutputType=Magnitude  PSBequivalent=0
  c : spsVoltageMeasurementLib/Voltage Measurement  Tag=PoWeRsYsTeMmEaSuReMeNt  PhasorSimulation=off  OutputType=Magnitude  PSBequivalent=0
  A : PMIOPort  Side=Left
  B : PMIOPort  Port=2  Side=Left
  C : PMIOPort  Port=3  Side=Left
  Vph : Outport  VectorParamsAs1DForOutWhenUnconnected=off
  VL-L : Outport  Port=2  VectorParamsAs1DForOutWhenUnconnected=off
  VL-L_rms : Outport  Port=3  VectorParamsAs1DForOutWhenUnconnected=off
  Vph_rms : Outport  Port=4  VectorParamsAs1DForOutWhenUnconnected=off
  wires:
  a/1 -> Mux7/1, Vab5/1
  b/1 -> Mux7/2, Vab1/1
  c/1 -> Mux7/3, Vab2/1
  Mux7/1 -> Vph/1
  Vab/1 -> Mux1/1
  Vbc/1 -> Mux1/2
  Vca/1 -> Mux1/3
  Mux1/1 -> Vab3/1, VL-L/1
  Vab5/1 -> Mux2/1
  Vab1/1 -> Mux2/2
  Vab2/1 -> Mux2/3
  Mux2/1 -> Vph_rms/1
  Vab3/1 -> VL-L_rms/1
  connections:
  Ground4/LConn1 -- c/LConn2 -- b/LConn2 -- a/LConn2
  A/RConn1 -- a/LConn1 -- Vab/LConn1 -- Vca/LConn2
  B/RConn1 -- b/LConn1 -- Vab/LConn2 -- Vbc/LConn1
  C/RConn1 -- c/LConn1 -- Vbc/LConn2 -- Vca/LConn1

== system Model_14Bus_Microgrid_paper_Latam/Subsystem3/Convertidor bidireccional 1.2 300 (DC) // 150 V (AC) P_nom 3kW/Control of Inverter ==
  note: VL-L rms_2
  note: Primary control
  note: Control of Inverter
  Means2 : Inport
  Bus Selector : BusSelector  OutputSignals=signal1,signal2,signal3,signal4
  Discrete PWM Generator1 : Subsystem  AncestorBlock=|  DialogController=POWERSYS.PowerSysDialog  mask(Discrete PWM Generator){GeneratorMode=3-arm  bridge (6 pulses), Fc=4000, Ts=Ts_Power, Internal=off, mIndex=0.99, Freq=60, Phase=0}
      | powerlib_extras/Discrete 
      | Control Blocks/Discrete
      | PWM Generator
      mask prompts: GeneratorMode "Generator Mode"; Fc "Carrier frequency (Hz):"; Ts "Sample time:"; Internal "Internal generation of modulating signal(s)"; mIndex "Modulation index  (0<m<1) :"; Freq "Frequency of output voltage (Hz)"; Phase "Phase of output voltage (degrees)"
      mask help:
      | This discrete block generates pulses for carrier-based PWM (Pulse Width Modulation), self-commutated IGBTs,GTOs or FETs bridges.
      |
      | Depending on the number of bridge arms selected in the "Generator Mode" parameter, the block can be used either for single-phase or three-phase PWM control.
      mask init: same as Model_14Bus_Microgrid_paper_Latam/Subsystem1/Convertidor bidireccional 1.1 300 (DC) // 150 V (AC) P_nom 3kW/Control of Inverter/Discrete PWM Generator1
      settings: LibrarySourceBlock=|
      | powerlib_extras/Discrete
      | Control Blocks/Discrete
      | PWM Generator
      mask Help:
      | The output pulses are a vector (with values=0 or 1). Depending on the selected "Generator Mode", the output vector contains:
      | For a 1-arm  bridge: Two pulses. Pulse 1 is for the upper switch and pulse 2 is for the lower switch.
      | For a 2-arm  bridge: Four pulses. Pulses 1 and 3 are respectively for the upper switches of the first and second arm. Pulses 2 and 4 are for the lower switches.
      | For a 3-arm  bridge: Six pulses. Pulses 1,3 and 5 are respectively for the upper switches of the first,second and third arm. Pulses 2,4 and 6 are for the lower switches.
      | For double 3-arm bridges: Twelve pulses.The first six pulses (pulses 1 to 6) must be sent to the first 3-arm bridge and the last six (pulses 7 to 12) to the second 3-arm bridge.
      | 
      | By selecting "Internal generation" you can can control the modulation index m, frequency and phase of the output voltage  from the internal parameters (m, Freq and Phase). Otherwise, external signals are used for pulse generation. The width of the input vector must be 1 for single phase bridges ( 1-arm or 2-arm)  and 3 for 3-phase bridges  (single or double bridge).
      mask TypeOptions GeneratorMode: 1-arm  bridge (2 pulses) | 2-arm  bridge (4 pulses) | 3-arm  bridge (6 pulses) | Double 3-arm  bridges (12 pulses)
      mask Callback Internal: powericon('psbcallbacks',gcb,'Discrete PWM Generator',[]);
  MI Controller : Subsystem
  Unit Delay4 : UnitDelay  SampleTime=Ts_Power  HasFrameUpgradeWarning=on
  VL-L_2 : Scope  NumInputPorts=2
  Vph_rms_2 : Scope
  m2 : Scope
  m_2 : Scope
  Pulses : Outport  VectorParamsAs1DForOutWhenUnconnected=off
  wires:
  MI Controller/2(m) -> m_2/1
  Unit Delay4/1 -> Pulses/1
  Discrete PWM Generator1/1(Pulses) -> Unit Delay4/1
  MI Controller/1(Vabc_inv) -> Discrete PWM Generator1/1(Uref)
  Bus Selector/1 -> m2/1, MI Controller/1(Vabc)  "<signal1>"
  Bus Selector/2 -> VL-L_2/1  "<signal2>"
  Bus Selector/3 -> VL-L_2/2  "<signal3>"
  Bus Selector/4 -> Vph_rms_2/1  "<signal4>"
  Means2/1 -> Bus Selector/1

== system Model_14Bus_Microgrid_paper_Latam/Subsystem4/Subsystem5/  Arreglo FV 10.5 kW ==
  note: DC Bus
  note: 10.5 - kW  PV Array
      | 42 * SunTech STP - 250S-20 /Wd  (Nser=6 Npar=7)
  Irradiance : Inport
  Temp2 : Inport  Port=2
  PV Array : spsPVArrayLib/PV Array  Npar=7  Nser=6  PlotType=array @ 1000 W/m2 & specified temperatures  S_vec="[ 1000  250 ]"  Temp_C_vec="[0 25 50  ]"  ModuleName=User-defined  PlotWhenSelected=off  Pm=250.205  Ncell=96  Voc=37.4  Isc=8.63  Vm=30.7  Im=8.15  beta_Voc_pc=-0.34  alpha_Isc_pc=0.050  beta_Voc=-0.12716  alpha_Isc=0.004315  IL=8.6686  I0=1.3965e-10  nI=0.6105  Rsh=311.9016  Rs=0.26776  RobustModel=off  RobustCellTemperature=313.3991  BAL=on  Tc=Tc  Tfilter=5e-5
  + : PMIOPort  Tag=PMCPort  Side=Left
  - : PMIOPort  Tag=PMCPort  Port=2  Side=Left
  tag scope: m_PV=global
  wires:
  Temp2/1 -> PV Array/2
  Irradiance/1 -> PV Array/1
  PV Array/1 -> [m_PV]
  connections:
  PV Array/RConn1 -- +/RConn1
  PV Array/RConn2 -- -/RConn1

== system Model_14Bus_Microgrid_paper_Latam/Subsystem4/Subsystem5/Convertidor boost DC //CD 5 kHz - 300V  ==
  note: DC_PV Bus
  note: DC bus Bus
  note: 5 kHz - 300V
      | Boost Converter
  note: 10.5-kW Grid-Connected PV Array (Detailed Model)
  " " : Subsystem  mask(Boost Control - MPPT){fc=5000, T_MPPT=200e-6, Dinit=0.25}
      mask prompts: fc "PWM switching frequency (Hz)"; T_MPPT "Time window used by MPPT control (s)"; Dinit "Initial value of duty cycle"
      mask Display: image('Icons\FPGA.png');
  C1 : spsSeriesRLCBranchLib/Series RLC Branch  LConnTagsString=__new0  RConnTagsString=__new0  BranchType=C  Resistance=1.0  Inductance=1.0  SetiL0=off  InitialCurrent=0  Capacitance=1200e-6  Setx0=off  InitialVoltage=0  Measurements=None
  C3 : spsSeriesRLCBranchLib/Series RLC Branch  LConnTagsString=__new0  RConnTagsString=__new0  BranchType=C  Resistance=1.0  Inductance=1.0  SetiL0=off  InitialCurrent=0  Capacitance=100e-6  Setx0=off  InitialVoltage=0  Measurements=Branch voltage
  Current Measurement1 : spsCurrentMeasurementLib/Current Measurement  PhasorSimulation=off  OutputType=Complex  PSBequivalent=0
  Current Measurement2 : spsCurrentMeasurementLib/Current Measurement  PhasorSimulation=off  OutputType=Complex  PSBequivalent=0
  Diode1 : spsDiodeLib/Diode  Ron=1e-4  Lon=0  Vf=0  IC=0  UseSnubber=off  Rs=inf  Cs=inf  Measurements=off
  Display{2..4,6} (4 alike) : Display
  IGBT1 : spsIGBTLib/IGBT  Ron=0.001  Lon=0  Vf=0  Tf=0  Tt=0  IC=0  Rs=1e5  Cs=inf  Measurements=off
  L1 : spsSeriesRLCBranchLib/Series RLC Branch  LConnTagsString=__new0  RConnTagsString=__new0  BranchType=RL  Resistance=0.005  Inductance=9e-3  SetiL0=off  InitialCurrent=0  Capacitance=1e-6  Setx0=off  InitialVoltage=0  Measurements=None
  Mean : spsMeanLib/Mean  Freq=10  Vinit=0  Ts=0
  Mean1 : spsMeanLib/Mean  Freq=10  Vinit=0  Ts=0
  Product : Product
  Step : Step  Time=0  SampleTime=0
  "Vdc " : spsVoltageMeasurementLib/Voltage Measurement  Tag=PoWeRsYsTeMmEaSuReMeNt  PhasorSimulation=off  OutputType=Magnitude  PSBequivalent=0
  Vdc 1 : spsVoltageMeasurementLib/Voltage Measurement  Tag=PoWeRsYsTeMmEaSuReMeNt  PhasorSimulation=off  OutputType=Magnitude  PSBequivalent=0
  B + : PMIOPort  Side=Right
  + : PMIOPort  Port=2  Side=Left
  - : PMIOPort  Port=3  Side=Left
  B - : PMIOPort  Port=4  Side=Right
  tag scope: I_DC_bus_PV=global, V_DC_bus_PV=global, g_boost_PV=global
  wires:
  [I_PV] -> " "/2(I_PV)
  " "/1(Pulses) -> Product/2
  [V_PV] -> " "/1(V_PV)
  Step/1 -> Product/1
  Current Measurement2/1 -> Mean1/1
  Mean/1 -> Display6/1
  Current Measurement1/1 -> [I_DC_bus_PV], Mean/1
  "Vdc "/1 -> Display3/1, [V_DC_bus_PV]
  Product/1 -> [g_boost_PV]
  [g_boost_PV] -> IGBT1/1
  Vdc 1/1 -> Display4/1
  Mean1/1 -> Display2/1
  connections:
  Current Measurement2/RConn1 -- Vdc 1/LConn1 -- L1/LConn1 -- C3/LConn1
  C3/RConn1 -- -/RConn1 -- C1/RConn1 -- "Vdc "/LConn2 -- IGBT1/RConn1 -- B -/RConn1 -- Vdc 1/LConn2
  IGBT1/LConn1 -- Diode1/LConn1 -- L1/RConn1
  B +/RConn1 -- Current Measurement2/LConn1
  +/RConn1 -- Current Measurement1/RConn1
  C1/LConn1 -- Current Measurement1/LConn1 -- Diode1/RConn1 -- "Vdc "/LConn1

== system Model_14Bus_Microgrid_paper_Latam/Subsystem4/Subsystem5/Resource1 ==
  note: http://calculationsolar.com/blog/?cat=2
  Constant1 : Constant  Value=max_min
  Irradiance (W/m^2) : Display
      settings: Format=bank  Decimation=1000
  Irradiance Temp Demand Max : Subsystem  Tag=STV Subsys  LoadFcn=sigbuilder_block('load');  StartFcn=sigbuilder_block('start');  StopFcn=sigbuilder_block('stop');  ClipboardFcn=sigbuilder_block('clipboard');  mask(Sigbuilder block){tuvar=[0:10]}
      mask help: Sigbuilder GUI
      mask init:
      | if ~strcmp(get_param(bdroot(gcbh),'SimulationStatus'),'stopped') tuvar = sigbuilder_block('maskInit'); end
      settings: CopyFcn=sigbuilder_block('copy');  DeleteFcn=sigbuilder_block('delete');  ModelCloseFcn=sigbuilder_block('modelClose');  PreSaveFcn=sigbuilder_block('preSave');  PauseFcn=sigbuilder_block('pause')  ContinueFcn=sigbuilder_block('continue')  NameChangeFcn=sigbuilder_block('namechange');  OpenFcn=sigbuilder_block('open',[0 30 1024.5 488.25 ]);  CloseFcn=sigbuilder_block('close');
      mask Display: plot(0, 0, 100, 100,[2, 2, 32, 32, 2], [68, 8, 8, 68, 68],[32, 2], [38, 38], [32, 19, 2],[53, 60, 44], [32, 17, 17, 2],[16, 16, 31, 31]);txt = getActiveGroup(gcbh);text(2, 100, txt,'verticalAlignment', 'top');
  Irradiance MIn Demand : Constant  Value=0
  Switch2 : Switch  Criteria=u2 > Threshold  SaturateOnIntegerOverflow=off  InputSameDT=off
  Temperature (deg. C) : Display
      settings: Format=bank  Decimation=1000
  Temp : Outport  VectorParamsAs1DForOutWhenUnconnected=off
  Ir : Outport  Port=2  VectorParamsAs1DForOutWhenUnconnected=off
  wires:
  Irradiance Temp Demand Max/1(Ir) -> Switch2/1, Irradiance (W/m^2)/1
  Irradiance Temp Demand Max/2(Temp) -> Temp/1, Temperature (deg. C)/1
  Irradiance MIn Demand/1 -> Switch2/3
  Constant1/1 -> Switch2/2
  Switch2/1 -> Ir/1  "Radiación (kW/m2)"

== system Model_14Bus_Microgrid_paper_Latam/Aerogenerador/PMSG Wind Turbine1/Control/Crow bar Protection ==
  Vdc_V : Inport
  Relay : Relay  OnSwitchValue=1500  OffSwitchValue=1300
  Pulses_crow_bar : Outport
  wires:
  Relay/1 -> Pulses_crow_bar/1
  Vdc_V/1 -> Relay/1

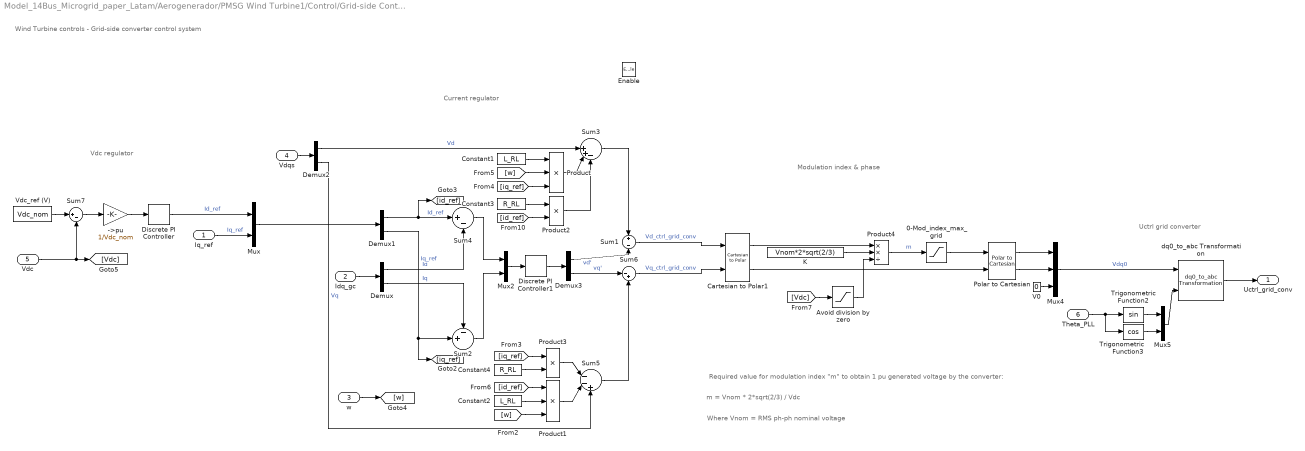
== system Model_14Bus_Microgrid_paper_Latam/Aerogenerador/PMSG Wind Turbine1/Control/Grid-side Controls ==
  note: Uctrl grid converter
  note: Modulation index & phase
  note: Current regulator
  note: Vdc regulator
  note: Required value for modulation index "m" to obtain 1 pu generated voltage by the converter:
  note: m = Vnom * 2*sqrt(2/3) / Vdc
  note: Where Vnom = RMS ph-ph nominal voltage
  note: Wind Turbine controls - Grid-side converter control system
  Iq_ref : Inport
  Idq_gc : Inport  Port=2
  w : Inport  Port=3
  Vdqs : Inport  Port=4
  Vdc : Inport  Port=5
  Theta_PLL : Inport  Port=6
  Enable : EnablePort
  ->pu : Gain  Gain=1/Vdc_nom
  0-Mod_index_max_grid : Saturate  UpperLimit=1.1  LowerLimit=0
  Avoid division by zero : Saturate  UpperLimit=inf  LowerLimit=1e-6
  Cartesian to Polar1 : simulink_extras/Transformations/Cartesian to Polar
  Constant1 : Constant  Value=L_RL
  Constant2 : Constant  Value=L_RL
  Constant3 : Constant  Value=R_RL
  Constant4 : Constant  Value=R_RL
  Demux{,1..3} (4 alike) : Demux  Outputs=2
      settings: DisplayOption=none
  Discrete PI Controller : powerlib_extras/Discrete  Control Blocks/Discrete PI Controller  Kp=8  Ki=400  Par_Limits=[1 -1]*1.2  Init=0  Ts=Ts
  Discrete PI Controller1 : powerlib_extras/Discrete  Control Blocks/Discrete PI Controller  Kp=0.83  Ki=5  Par_Limits=[1.0 -1.0] *1.1  Init=0  Ts=Ts
  K : Constant  Value=Vnom*2*sqrt(2/3)
  Mux : Mux  Inputs=2
  Mux2 : Mux  Inputs=2
  Mux4 : Mux  Inputs=3
  Mux5 : Mux  Inputs=2
  Polar to Cartesian : simulink_extras/Transformations/Polar to Cartesian
  Product : Product  Inputs=3  InputSameDT=on  SaturateOnIntegerOverflow=on  OutDataTypeStr=Inherit: Same as first input
  Product1 : Product  Inputs=3  InputSameDT=on  SaturateOnIntegerOverflow=on  OutDataTypeStr=Inherit: Same as first input
  Product2 : Product  InputSameDT=on  SaturateOnIntegerOverflow=on  OutDataTypeStr=Inherit: Same as first input
  Product3 : Product  InputSameDT=on  SaturateOnIntegerOverflow=on  OutDataTypeStr=Inherit: Same as first input
  Product4 : Product  Inputs=**/  InputSameDT=on  SaturateOnIntegerOverflow=on  OutDataTypeStr=Inherit: Same as first input
  Sum1 : Sum  Inputs=+-  InputSameDT=on  SaturateOnIntegerOverflow=on  OutDataTypeStr=Inherit: Same as first input
  Sum2 : Sum  Inputs=-+|  InputSameDT=on  SaturateOnIntegerOverflow=on  OutDataTypeStr=Inherit: Same as first input
  Sum3 : Sum  Inputs=||++-  InputSameDT=on  SaturateOnIntegerOverflow=on  OutDataTypeStr=Inherit: Same as first input
  Sum4 : Sum  Inputs=|+-  InputSameDT=on  SaturateOnIntegerOverflow=on  OutDataTypeStr=Inherit: Same as first input
  Sum5 : Sum  Inputs=|--+  InputSameDT=on  SaturateOnIntegerOverflow=on  OutDataTypeStr=Inherit: Same as first input
  Sum6 : Sum  Inputs=|-+  InputSameDT=on  SaturateOnIntegerOverflow=on  OutDataTypeStr=Inherit: Same as first input
  Sum7 : Sum  Inputs=|+-  InputSameDT=on  SaturateOnIntegerOverflow=on  OutDataTypeStr=Inherit: Same as first input
  Trigonometric Function2 : Trigonometry
  Trigonometric Function3 : Trigonometry  Operator=cos
  V0 : Constant  Value=0
  Vdc_ref (V) : Constant  Value=Vdc_nom
  dq0_to_abc Transformation : powerlib_extras/Measurements/dq0_to_abc Transformation
  Uctrl_grid_conv : Outport
  wires:
  Sum6/1 -> Cartesian to Polar1/2  "Vq_ctrl_grid_conv"
  Sum1/1 -> Cartesian to Polar1/1  "Vd_ctrl_grid_conv"
  dq0_to_abc Transformation/1 -> Uctrl_grid_conv/1
  Theta_PLL/1 -> Trigonometric Function2/1, Trigonometric Function3/1
  Mux4/1 -> dq0_to_abc Transformation/1  "Vdq0"
  Polar to Cartesian/2 -> Mux4/2
  Polar to Cartesian/1 -> Mux4/1
  V0/1 -> Mux4/3
  Trigonometric Function3/1 -> Mux5/2
  Trigonometric Function2/1 -> Mux5/1
  Mux5/1 -> dq0_to_abc Transformation/2
  [Vdc] -> Avoid division by zero/1
  Product4/1 -> 0-Mod_index_max_grid/1  "m"
  K/1 -> Product4/2
  Avoid division by zero/1 -> Product4/3
  Cartesian to Polar1/1 -> Product4/1
  0-Mod_index_max_grid/1 -> Polar to Cartesian/1
  Cartesian to Polar1/2 -> Polar to Cartesian/2
  Mux/1 -> Demux1/1
  Idq_gc/1 -> Demux/1
  w/1 -> [w]
  Constant2/1 -> Product1/2
  Discrete PI Controller1/1 -> Demux3/1
  Mux2/1 -> Discrete PI Controller1/1
  Demux2/1 -> Sum3/1  "Vd"
  Constant1/1 -> Product/1
  Vdqs/1 -> Demux2/1
  Demux/2 -> Sum2/1  "Iq"
  Demux/1 -> Sum4/2  "Id"
  Product/1 -> Sum3/2
  Constant3/1 -> Product2/1
  Constant4/1 -> Product3/2
  Product1/1 -> Sum5/2
  Demux2/2 -> Sum5/3  "Vq"
  Product2/1 -> Sum3/3
  Product3/1 -> Sum5/1
  Sum4/1 -> Mux2/1
  Sum2/1 -> Mux2/2
  [w] -> Product1/3
  [w] -> Product/2
  [iq_ref] -> Product/3
  [id_ref] -> Product2/2
  [iq_ref] -> Product3/1
  [id_ref] -> Product1/1
  Demux3/1 -> Sum1/2  "vd'"
  Demux3/2 -> Sum6/1  "vq'"
  Demux1/2 -> [iq_ref], Sum2/2  "Iq_ref"
  Demux1/1 -> Sum4/1, [id_ref]  "Id_ref"
  Sum3/1 -> Sum1/1
  Sum5/1 -> Sum6/2
  Discrete PI Controller/1 -> Mux/1  "Id_ref"
  Sum7/1 -> ->pu/1
  ->pu/1 -> Discrete PI Controller/1
  Vdc/1 -> [Vdc], Sum7/2
  Iq_ref/1 -> Mux/2  "Iq_ref"
  Vdc_ref (V)/1 -> Sum7/1
